simulink model "MASH_Derived"  (R2025b)
settings: Solver=VariableStepAuto  StartTime=0.0  StopTime=4.608  RelTol=1e-9
model workspace (MAT data in the model file):
  Delay_20 = [0 0 0]
  Delay_53 = [0 0 0]
  Delay_70 = [0 0 0]
  Delay_87 = [0 0 0]
  ENOB_20 = 14.7610440397
  ENOB_53 = 14.7608825493
  ENOB_70 = 14.7022390875
  ENOB_87 = 14.7022390875
  FUNDF_20 = [900.000005068 999.349381913]
  FUNDF_53 = [900.000005078 999.349381913]
  FUNDF_70 = [900.000004559 999.349381913]
  FUNDF_87 = [900.000004559 999.349381913]
  FUNDX_20 = [23.0527289443 -77.1427323486]
  FUNDX_53 = [23.0527291545 -77.1418515114]
  FUNDX_70 = [23.0527299683 -77.0677275157]
  FUNDX_87 = [23.0527299683 -77.0677275157]
  IMODF_20 = [800.829599918 nan]
  IMODF_53 = [800.8283682 nan]
  IMODF_70 = [800.868701953 nan]
  IMODF_87 = [800.868701953 nan]
  IMODX_20 = [-76.1327176352 nan]
  IMODX_53 = [-76.130863984 nan]
  IMODX_70 = [-76.3681290279 nan]
  IMODX_87 = [-76.3681290279 nan]
  NoiseFloor_20 = -89.9553424364
  NoiseFloor_53 = -89.9779075363
  NoiseFloor_70 = -90.20149126
  NoiseFloor_87 = -90.20149126
  OIP3_20 = nan
  OIP3_53 = nan
  OIP3_70 = nan
  OIP3_87 = nan
  SFDR_20 = 99.5065630611
  SFDR_53 = 99.5056824376
  SFDR_70 = 99.4315580441
  SFDR_87 = 99.4315580441
  SINAD_20 = 90.621485119
  SINAD_53 = 90.6205129467
  SINAD_70 = 90.267479307
  SINAD_87 = 90.267479307
  SNR_20 = 90.621485119
  SNR_53 = 90.6205129467
  SNR_70 = 90.267479307
  SNR_87 = 90.267479307
  THD_20 = -inf
  THD_53 = -inf
  THD_70 = -inf
  THD_87 = -inf
  delay_20 = [0 0 0]
  delay_53 = [0 0 0]
  delay_70 = [0 0 0]
  delay_87 = [0 0 0]
undefined symbols (not defined in the file): designMultirateFIR, dspblkCoreblockFVToolHelper, gcbh
libraries: msbAdcFoundation x8, msbAdcMeasurements x4, dspmlti4 x4
settings Model: Creator=The MathWorks, Inc.  LastModifiedBy=sohom
settings RTWCC: LargeConstantGeneration=WriteOnlyDNNConstantsToDataFiles

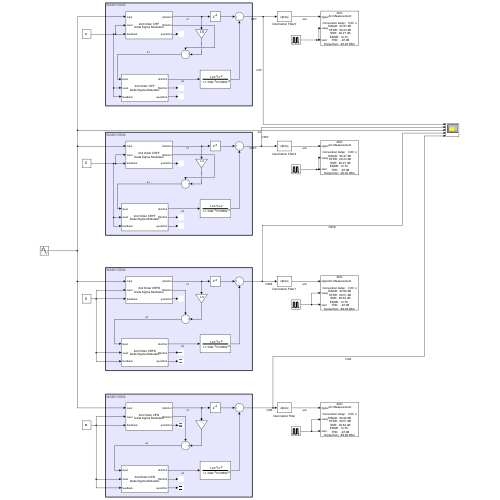
[thumbnail: Simulink's stored preview of the top-level diagram]
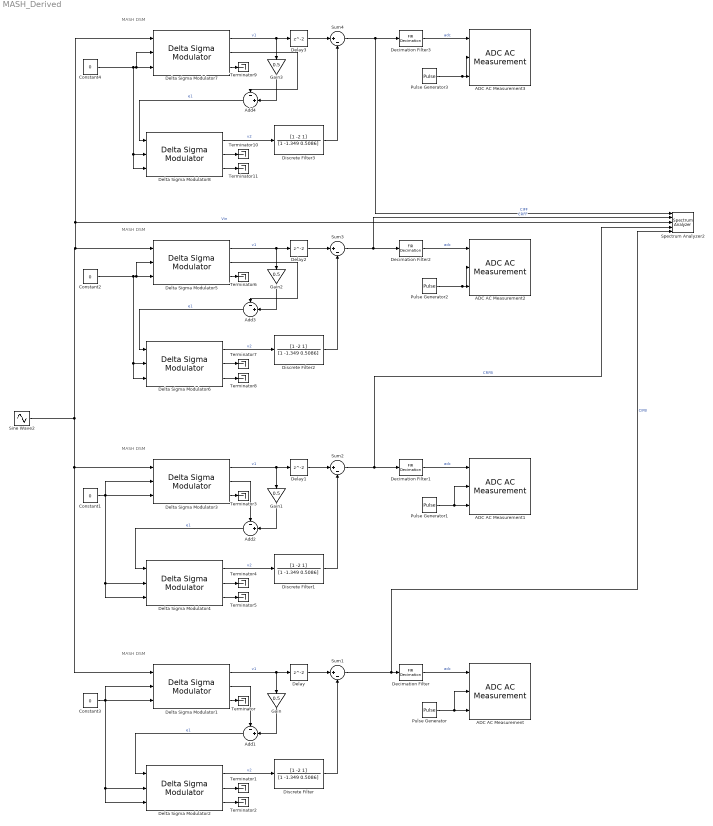
== system MASH_Derived ==
  note: MASH DSM
  note: MASH DSM
  note: MASH DSM
  note: MASH DSM
  ADC AC Measurement{,1..3} (4 alike) : msbAdcMeasurements/ADC AC Measurement  DistortionMeasurement=Harmonic  InputFrequency=900  Method=Welch (faster, potentially more leakage)  RBW=1.9531  AutoSetRBW=on  NBits=5  Frequency=2e3  HoldOffTime=0  OutputToWorkspace=on  VariableName=mash_ac_out  ShowSpectrum=off
  Add{1..4} (4 alike) : Sum  Inputs=-+|
  Constant{1..4} (4 alike) : Constant  Value=0
  Decimation Filter{,1..3} (4 alike) : dspmlti4/FIR Decimation  FilterSource=Auto  h=designMultirateFIR(1,2)  D=64  filtStruct=Direct form  FilterObject=FDECIM  framing=Allow multirate processing  AllowArbitraryInputLength=off  inputOffset=0  outputBufInitCond=0  roundingMode=Floor  overflowMode=off  firstCoeffDataTypeStr=Inherit: Same word length as input  firstCoeffMin=[]  firstCoeffMax=[]  firstCoeffLastDataTypeStr=Inherit: Same word length as input  outputDataTypeStr=Inherit: Same as accumulator  outputMin=[]  outputMax=[]  outputLastDataTypeStr=Inherit: Same as accumulator
      settings: LibrarySourceBlock=|
      | dsphdlsupportfiltering/FIR
      | Decimation
  Delay{,1..3} (4 alike) : Delay
  Delta Sigma Modulator1 : msbAdcFoundation/Delta Sigma Modulator  dsmArchitecture=CIFB  dsmOrder=2nd order  BandWidth=1000  OSR=64  SamplingFrequency=128000  NumberLevels=2  QuantizerOutput=-1:2:1  BoundaryPoints=[-1:1:1]  EnableDynamicRangeScaling=off  EnableCustomCoeff=off  a=[0.1601 0.6515]  g=[0.0000]  b=[0.1601 0.6515 1.0000]  c=[1.0000 1.0000]  OLgain=Inf  EnableNoise=off  thermalNoiseValue=200e-6  thermalNoiseUnit=Vrms  refResistance=50  wNoiseGain=0.0002  fcorner=1000  pNoiseGain=5e-06  ntfOptim=2: Optimized with at least one zero at band-center  passbandType=Lowpass  centerFrequency=0  EnableCustomHinf=off  Hinf=1.4  NTFflag=on  PZflag=off  STFflag=off  SNRflag=off  AppendFlag=off  ExportFlag=off
      link override Delta Sigma Modulator: LabelModeActiveChoice=2CIFB
      link override Noise: LabelModeActiveChoice=noNoise
  Delta Sigma Modulator2 : msbAdcFoundation/Delta Sigma Modulator  dsmArchitecture=CIFB  dsmOrder=2nd order  BandWidth=1000  OSR=64  SamplingFrequency=128000  NumberLevels=2  QuantizerOutput=-1:2:1  BoundaryPoints=[-1:1:1]  EnableDynamicRangeScaling=off  EnableCustomCoeff=off  a=[0.1601 0.6515]  g=[0.0000]  b=[0.1601 0.6515 1.0000]  c=[1.0000 1.0000]  OLgain=Inf  EnableNoise=off  thermalNoiseValue=200e-6  thermalNoiseUnit=Vrms  refResistance=50  wNoiseGain=0.0002  fcorner=1000  pNoiseGain=5e-06  ntfOptim=2: Optimized with at least one zero at band-center  passbandType=Lowpass  centerFrequency=0  EnableCustomHinf=off  Hinf=1.4  NTFflag=on  PZflag=off  STFflag=off  SNRflag=off  AppendFlag=off  ExportFlag=off
      link override Delta Sigma Modulator: LabelModeActiveChoice=2CIFB
      link override Noise: LabelModeActiveChoice=noNoise
  Delta Sigma Modulator3 : msbAdcFoundation/Delta Sigma Modulator  dsmArchitecture=CRFB  dsmOrder=2nd order  BandWidth=1000  OSR=64  SamplingFrequency=128000  NumberLevels=2  QuantizerOutput=-1:2:1  BoundaryPoints=[-1:1:1]  EnableDynamicRangeScaling=off  EnableCustomCoeff=off  a=[0.1601 0.4914]  g=[0.0000]  b=[0.1601 0.4914 1.0000]  c=[1.0000 1.0000]  OLgain=Inf  EnableNoise=off  thermalNoiseValue=200e-6  thermalNoiseUnit=Vrms  refResistance=50  wNoiseGain=0.0002  fcorner=1000  pNoiseGain=5e-06  ntfOptim=2: Optimized with at least one zero at band-center  passbandType=Lowpass  centerFrequency=0  EnableCustomHinf=off  Hinf=1.4  NTFflag=on  PZflag=off  STFflag=off  SNRflag=off  AppendFlag=off  ExportFlag=off
      link override Delta Sigma Modulator: LabelModeActiveChoice=2CRFB
      link override Noise: LabelModeActiveChoice=noNoise
  Delta Sigma Modulator4 : msbAdcFoundation/Delta Sigma Modulator  dsmArchitecture=CRFB  dsmOrder=2nd order  BandWidth=1000  OSR=64  SamplingFrequency=128000  NumberLevels=2  QuantizerOutput=-1:2:1  BoundaryPoints=[-1:1:1]  EnableDynamicRangeScaling=off  EnableCustomCoeff=off  a=[0.1601 0.4914]  g=[0.0000]  b=[0.1601 0.4914 1.0000]  c=[1.0000 1.0000]  OLgain=Inf  EnableNoise=off  thermalNoiseValue=200e-6  thermalNoiseUnit=Vrms  refResistance=50  wNoiseGain=0.0002  fcorner=1000  pNoiseGain=5e-06  ntfOptim=2: Optimized with at least one zero at band-center  passbandType=Lowpass  centerFrequency=0  EnableCustomHinf=off  Hinf=1.4  NTFflag=on  PZflag=off  STFflag=off  SNRflag=off  AppendFlag=off  ExportFlag=off
      link override Delta Sigma Modulator: LabelModeActiveChoice=2CRFB
      link override Noise: LabelModeActiveChoice=noNoise
  Delta Sigma Modulator5 : msbAdcFoundation/Delta Sigma Modulator  dsmArchitecture=CRFF  dsmOrder=2nd order  BandWidth=1000  OSR=64  SamplingFrequency=128000  NumberLevels=2  QuantizerOutput=-1:2:1  BoundaryPoints=[-1:1:1]  EnableDynamicRangeScaling=off  EnableCustomCoeff=off  a=[0.4914 0.1601]  g=[0.0000]  b=[1.0000 0.0000 1.0000]  c=[1.0000 1.0000]  OLgain=Inf  EnableNoise=off  thermalNoiseValue=200e-6  thermalNoiseUnit=Vrms  refResistance=50  wNoiseGain=0.0002  fcorner=1000  pNoiseGain=5e-06  ntfOptim=2: Optimized with at least one zero at band-center  passbandType=Lowpass  centerFrequency=0  EnableCustomHinf=off  Hinf=1.4  NTFflag=on  PZflag=off  STFflag=off  SNRflag=off  AppendFlag=off  ExportFlag=off
      link override Delta Sigma Modulator: LabelModeActiveChoice=2CRFF
      link override Noise: LabelModeActiveChoice=noNoise
  Delta Sigma Modulator6 : msbAdcFoundation/Delta Sigma Modulator  dsmArchitecture=CRFF  dsmOrder=2nd order  BandWidth=1000  OSR=64  SamplingFrequency=128000  NumberLevels=2  QuantizerOutput=-1:2:1  BoundaryPoints=[-1:1:1]  EnableDynamicRangeScaling=off  EnableCustomCoeff=off  a=[0.4914 0.1601]  g=[0.0000]  b=[1.0000 0.0000 1.0000]  c=[1.0000 1.0000]  OLgain=Inf  EnableNoise=off  thermalNoiseValue=200e-6  thermalNoiseUnit=Vrms  refResistance=50  wNoiseGain=0.0002  fcorner=1000  pNoiseGain=5e-06  ntfOptim=2: Optimized with at least one zero at band-center  passbandType=Lowpass  centerFrequency=0  EnableCustomHinf=off  Hinf=1.4  NTFflag=on  PZflag=off  STFflag=off  SNRflag=off  AppendFlag=off  ExportFlag=off
      link override Delta Sigma Modulator: LabelModeActiveChoice=2CRFF
      link override Noise: LabelModeActiveChoice=noNoise
  Delta Sigma Modulator7 : msbAdcFoundation/Delta Sigma Modulator  dsmArchitecture=CIFF  dsmOrder=2nd order  BandWidth=1000  OSR=64  SamplingFrequency=128000  NumberLevels=2  QuantizerOutput=-1:2:1  BoundaryPoints=[-1:1:1]  EnableDynamicRangeScaling=off  EnableCustomCoeff=off  a=[0.6515 0.1601]  g=[0.0000]  b=[1.0000 0.0000 1.0000]  c=[1.0000 1.0000]  OLgain=Inf  EnableNoise=off  thermalNoiseValue=200e-6  thermalNoiseUnit=Vrms  refResistance=50  wNoiseGain=0.0002  fcorner=1000  pNoiseGain=5e-06  ntfOptim=2: Optimized with at least one zero at band-center  passbandType=Lowpass  centerFrequency=0  EnableCustomHinf=off  Hinf=1.4  NTFflag=on  PZflag=off  STFflag=off  SNRflag=off  AppendFlag=off  ExportFlag=off
      link override Delta Sigma Modulator: LabelModeActiveChoice=2CIFF
      link override Noise: LabelModeActiveChoice=noNoise
  Delta Sigma Modulator8 : msbAdcFoundation/Delta Sigma Modulator  dsmArchitecture=CIFF  dsmOrder=2nd order  BandWidth=1000  OSR=64  SamplingFrequency=128000  NumberLevels=2  QuantizerOutput=-1:2:1  BoundaryPoints=[-1:1:1]  EnableDynamicRangeScaling=off  EnableCustomCoeff=off  a=[0.6515 0.1601]  g=[0.0000]  b=[1.0000 0.0000 1.0000]  c=[1.0000 1.0000]  OLgain=Inf  EnableNoise=off  thermalNoiseValue=200e-6  thermalNoiseUnit=Vrms  refResistance=50  wNoiseGain=0.0002  fcorner=1000  pNoiseGain=5e-06  ntfOptim=2: Optimized with at least one zero at band-center  passbandType=Lowpass  centerFrequency=0  EnableCustomHinf=off  Hinf=1.4  NTFflag=on  PZflag=off  STFflag=off  SNRflag=off  AppendFlag=off  ExportFlag=off
      link override Delta Sigma Modulator: LabelModeActiveChoice=2CIFF
      link override Noise: LabelModeActiveChoice=noNoise
  Discrete Filter{,1..3} (4 alike) : DiscreteFilter  LoadFcn=dspblkCoreblockFVToolHelper(gcbh,'load');  Numerator=[1 -2 1]  Denominator=[1 -1.349 0.5086]
      settings: CopyFcn=dspblkCoreblockFVToolHelper(gcbh,'copy');  DeleteFcn=dspblkCoreblockFVToolHelper(gcbh,'close');  ModelCloseFcn=dspblkCoreblockFVToolHelper(gcbh,'close');  PreSaveFcn=dspblkCoreblockFVToolHelper(gcbh,'presave');  PostSaveFcn=dspblkCoreblockFVToolHelper(gcbh,'postsave');  CloseFcn=dspblkCoreblockFVToolHelper(gcbh,'close');
  Gain{,1..3} (4 alike) : Gain  Gain=0.5
  Pulse Generator{,1..3} (4 alike) : DiscretePulseGenerator  PulseType=Time based  Period=1/2e3  PulseWidth=50
  Sine Wave2 : Sin  Amplitude=0.7  Frequency=2*pi*0.9e3  Phase=pi  SampleTime=1/128e3
  Spectrum Analyzer2 : SpectrumAnalyzer  NumInputPorts=5  WindowPosition=[42.000000,33.000000,1209.000000,591.000000,]  ScopeFrameLocation=window  SpectrumType=Power density  SampleRate=44.1e3  PlotAsTwoSidedSpectrum=off  FrequencyScale=Log  StartFrequency=20  StopFrequency=20e3  SpectrumUnits=dBm/Hz  YLimits=[-86.5536 13.926]  ShowLegend=on
  Sum{1..4} (4 alike) : Sum  Inputs=|+-
  Terminator{,1..11} (12 alike) : Terminator
  wires:
  Delta Sigma Modulator1/1 -> Gain/1, Delay/1  "v1"
  Delay/1 -> Sum1/1
  Constant3/1 -> Delta Sigma Modulator1/2, Delta Sigma Modulator2/2, Delta Sigma Modulator2/3, Delta Sigma Modulator1/3
  Delta Sigma Modulator2/2 -> Terminator1/1
  Sum1/1 -> Spectrum Analyzer2/5, Decimation Filter/1  "CIFB"
  Delta Sigma Modulator1/2 -> Add1/1
  Delta Sigma Modulator1/3 -> Terminator/1
  Delta Sigma Modulator2/3 -> Terminator2/1
  Gain/1 -> Add1/2
  Pulse Generator/1 -> ADC AC Measurement/3, ADC AC Measurement/2
  Decimation Filter/1 -> ADC AC Measurement/1  "adc"
  Delta Sigma Modulator2/1 -> Discrete Filter/1  "v2"
  Discrete Filter/1 -> Sum1/2
  Add1/1 -> Delta Sigma Modulator2/1  "e1"
  Constant1/1 -> Delta Sigma Modulator3/2, Delta Sigma Modulator4/2, Delta Sigma Modulator4/3, Delta Sigma Modulator3/3
  Decimation Filter1/1 -> ADC AC Measurement1/1  "adc"
  Gain1/1 -> Add2/2
  Delta Sigma Modulator3/2 -> Add2/1
  Discrete Filter1/1 -> Sum2/2
  Delay1/1 -> Sum2/1
  Delta Sigma Modulator3/3 -> Terminator3/1
  Pulse Generator1/1 -> ADC AC Measurement1/3, ADC AC Measurement1/2
  Add2/1 -> Delta Sigma Modulator4/1  "e1"
  Delta Sigma Modulator4/2 -> Terminator4/1
  Delta Sigma Modulator3/1 -> Gain1/1, Delay1/1  "v1"
  Delta Sigma Modulator4/1 -> Discrete Filter1/1  "v2"
  Delta Sigma Modulator4/3 -> Terminator5/1
  Sum2/1 -> Spectrum Analyzer2/4, Decimation Filter1/1  "CRFB"
  Sum3/1 -> Decimation Filter2/1, Spectrum Analyzer2/2  "CRFF"
  Delta Sigma Modulator6/3 -> Terminator8/1
  Delta Sigma Modulator5/1 -> Gain2/1, Delay2/1  "v1"
  Delay2/1 -> Sum3/1
  Discrete Filter2/1 -> Sum3/2
  Add3/1 -> Delta Sigma Modulator6/1  "e1"
  Delta Sigma Modulator6/2 -> Terminator7/1
  Pulse Generator2/1 -> ADC AC Measurement2/3, ADC AC Measurement2/2
  Gain2/1 -> Add3/2
  Delta Sigma Modulator5/2 -> Add3/1
  Delta Sigma Modulator5/3 -> Terminator6/1
  Delta Sigma Modulator6/1 -> Discrete Filter2/1  "v2"
  Decimation Filter2/1 -> ADC AC Measurement2/1  "adc"
  Constant2/1 -> Delta Sigma Modulator6/2, Delta Sigma Modulator6/3, Delta Sigma Modulator5/2, Delta Sigma Modulator5/3
  Sum4/1 -> Spectrum Analyzer2/1, Decimation Filter3/1  "CIFF"
  Delta Sigma Modulator8/3 -> Terminator11/1
  Delta Sigma Modulator7/1 -> Gain3/1, Delay3/1  "v1"
  Delay3/1 -> Sum4/1
  Discrete Filter3/1 -> Sum4/2
  Add4/1 -> Delta Sigma Modulator8/1  "e1"
  Delta Sigma Modulator8/2 -> Terminator10/1
  Pulse Generator3/1 -> ADC AC Measurement3/3, ADC AC Measurement3/2
  Gain3/1 -> Add4/2
  Delta Sigma Modulator7/2 -> Add4/1
  Delta Sigma Modulator7/3 -> Terminator9/1
  Delta Sigma Modulator8/1 -> Discrete Filter3/1  "v2"
  Decimation Filter3/1 -> ADC AC Measurement3/1  "adc"
  Constant4/1 -> Delta Sigma Modulator8/2, Delta Sigma Modulator8/3, Delta Sigma Modulator7/2, Delta Sigma Modulator7/3
  Sine Wave2/1 -> Delta Sigma Modulator1/1, Delta Sigma Modulator3/1, Spectrum Analyzer2/3, Delta Sigma Modulator7/1, Delta Sigma Modulator5/1  "Vin"
